simulink model "MotorModel"  (Simulink 6.5)
settings: Solver=FixedStepDiscrete  StartTime=0.0  StopTime=1  FixedStep=0.01  RelTol=1e-3
libraries: c28xdmclib x1, simulink x1
settings Model: Creator=Phono  LastModifiedBy=jfaing

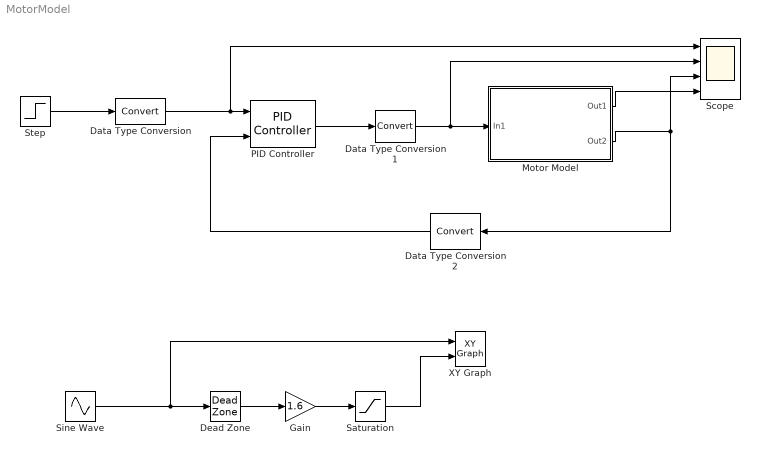
== system MotorModel ==
  Data Type Conversion : DataTypeConversion  OutDataTypeMode=Specify via dialog  OutDataType=sfix(32)  OutScaling=2^-15  RndMeth=Nearest  SampleTime=0.01  SaturateOnIntegerOverflow=on
  Data Type Conversion1 : DataTypeConversion  OutDataTypeMode=double  OutDataType=sfix(32)  OutScaling=2^-15  RndMeth=Nearest  SaturateOnIntegerOverflow=on
  Data Type Conversion2 : DataTypeConversion  Orientation=left  OutDataTypeMode=Specify via dialog  OutDataType=sfix(32)  OutScaling=2^-15  RndMeth=Nearest  SaturateOnIntegerOverflow=on
  Dead Zone : DeadZone  LowerValue=-6  UpperValue=6  SampleTime=0.01  SaturateOnIntegerOverflow=on
  Gain : Gain  Gain=1.6
  Motor Model : Subsystem
  PID Controller : c28xdmclib/PID Controller  proportionalGain=0.2  integralGain=0.9  correctionGain=0.6  derivativeGain=1.2  minOutput=6  maxOutput=15
  Saturation : Saturate  UpperLimit=15  LowerLimit=0  SampleTime=0.01
  Scope : Scope  NumInputPorts=4
      settings: YMin=-5~-5~-5~-5  YMax=5~5~5~5
  Sine Wave : Sin  Amplitude=30  SampleTime=0.01
  Step : Step  Time=0  After=800  SampleTime=0
  XY Graph : simulink/Sinks/XY Graph  SystemSampleTime=-1  xmin=0  xmax=30  ymin=0  ymax=30  st=0.01
  wires:
  Motor Model/2(Out2) -> Data Type Conversion2/1, Scope/3
  Step/1 -> Data Type Conversion/1
  Data Type Conversion/1 -> PID Controller/1, Scope/1
  PID Controller/1 -> Data Type Conversion1/1
  Data Type Conversion1/1 -> Scope/2, Motor Model/1(In1)
  Data Type Conversion2/1 -> PID Controller/2
  Dead Zone/1 -> Gain/1
  Sine Wave/1 -> Dead Zone/1, XY Graph/1
  Saturation/1 -> XY Graph/2
  Gain/1 -> Saturation/1
  Motor Model/1(Out1) -> Scope/4

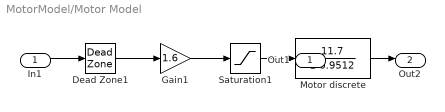
== system MotorModel/Motor Model ==
  In1 : Inport
  Dead Zone1 : DeadZone  LowerValue=-6  UpperValue=6  SampleTime=0.01  SaturateOnIntegerOverflow=on
  Gain1 : Gain  Gain=1.6
  Motor discrete : DiscreteTransferFcn  Numerator=[11.7]  Denominator=[1 -0.9512]  SampleTime=0.01
  Saturation1 : Saturate  UpperLimit=15  LowerLimit=0  SampleTime=0.01
  Out1 : Outport
  Out2 : Outport  Port=2
  wires:
  Dead Zone1/1 -> Gain1/1
  Gain1/1 -> Saturation1/1
  Saturation1/1 -> Motor discrete/1, Out1/1
  In1/1 -> Dead Zone1/1
  Motor discrete/1 -> Out2/1
